simulink model "servo"  (R2018a)
settings: Solver=VariableStepAuto  StartTime=0.0  StopTime=T  RelTol=1e-3
values from neighbouring files (symbols this model uses):
  C0 = 0.024    [asserv_ge2M.m]
  f = 5.06e-5    (= 5.06e-05)    [asserv_ge2M.m]
  Ghelice = 28.35*h*D^3*10^-10*Sgouv    [asserv_ge2M.m]
  Gredu = 1    [asserv_ge2M.m]
  Gservo = 1    [asserv_ge2M.m]
  J = 8.3e-5    (= 8.3e-05)    [asserv_ge2M.m]
  Kphi = 0.127    [asserv_ge2M.m]
  KpS = 1    [asserv_ge2M.m]
  L = 2.2e-3    (= 0.0022)    [asserv_ge2M.m]
  R = 1.52    [asserv_ge2M.m]
  Step = pi    (= 3.14159265359)    [asserv_ge2M.m]
  Vit = 10000/60    (= 166.666666667)    [asserv_ge2M.m]
libraries: simulink x1
settings Model: Creator=xoxox  LastModifiedBy=xoxox

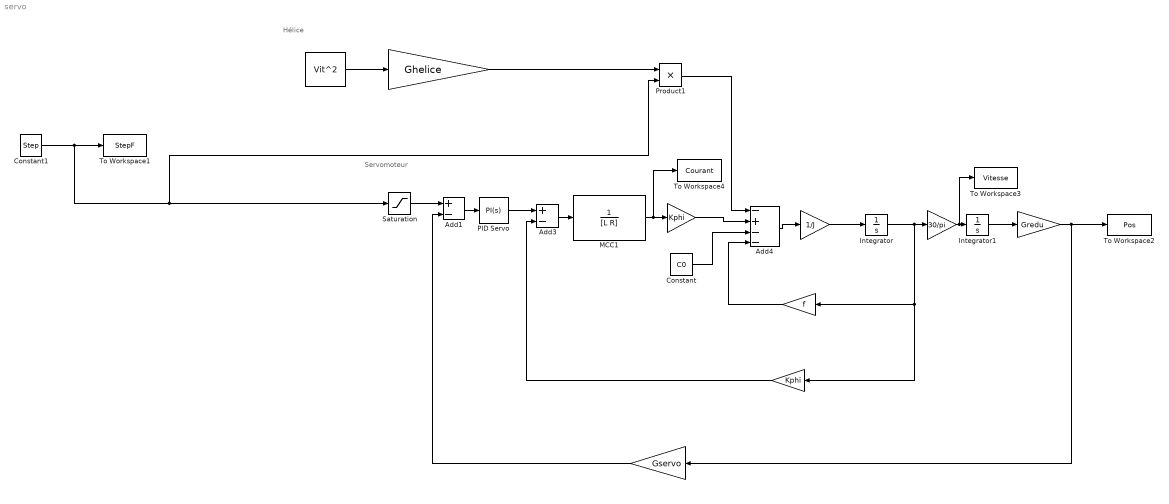
== system servo ==
  note: Servomoteur
  note: Hélice
  " " : Gain  Gain=Kphi
  " " : Gain  Gain=Gservo
  " " : Gain  Gain=Gredu
  "  " : Gain  Gain=Kphi
  " " : Constant  Value=Vit^2
  " " : Gain  Gain=1/J
  " " : Gain  Gain=Ghelice
  "     " : Gain  Gain=f
  " " : Gain  Gain=30/pi
  Add1 : Sum  Inputs=+-
  Add3 : Sum  Inputs=+-
  Add4 : Sum  Inputs=-+--
  Constant : Constant  Value=C0
  Constant1 : Constant  Value=Step
  Integrator : Integrator
  Integrator1 : Integrator
  MCC1 : TransferFcn  Denominator=[L R]
  PID Servo : simulink/Continuous/PID Controller  Controller=PI  TimeDomain=Continuous-time  SampleTime=-1  IntegratorMethod=Forward Euler  FilterMethod=Forward Euler  Form=Parallel  UseFilter=on  ControllerParametersSource=internal  P=KpS  I=0  D=0  N=100  InitialConditionSource=internal  InitialConditionForIntegrator=0  InitialConditionForFilter=0  ExternalReset=none  LimitOutput=off  UpperSaturationLimit=inf  LowerSaturationLimit=-inf  LinearizeAsGain=on  AntiWindupMode=none  Kb=1  TrackingMode=off  Kt=1  PParamMin=[]  PParamMax=[]  IParamMin=[]  IParamMax=[]  DParamMin=[]  DParamMax=[]  NParamMin=[]  NParamMax=[]  KbParamMin=[]  KbParamMax=[]  KtParamMin=[]  KtParamMax=[]  POutMin=[]  POutMax=[]  IOutMin=[]  IOutMax=[]  DOutMin=[]  DOutMax=[]  NOutMin=[]  NOutMax=[]  KbOutMin=[]  KbOutMax=[]  KtOutMin=[]  KtOutMax=[]  IntegratorOutMin=[]  IntegratorOutMax=[]  FilterOutMin=[]  FilterOutMax=[]  SumOutMin=[]  SumOutMax=[]  SumI1OutMin=[]  SumI1OutMax=[]  SumI2OutMin=[]  SumI2OutMax=[]  SumI3OutMin=[]  SumI3OutMax=[]  SumDOutMin=[]  SumDOutMax=[]  SaturationOutMin=[]  SaturationOutMax=[]  IntegratorContinuousStateAttributes=''  IntegratorStateMustResolveToSignalObject=off  IntegratorRTWStateStorageClass=Auto  FilterContinuousStateAttributes=''  FilterStateMustResolveToSignalObject=off  FilterRTWStateStorageClass=Auto  DifferentiatorICPrevScaledInput=0  DifferentiatorOutMin=[]  DifferentiatorOutMax=[]  FilterDiffOutCoefMin=[]  FilterDiffOutCoefMax=[]  SumDenOutMin=[]  SumDenOutMax=[]  SumNumOutMin=[]  SumNumOutMax=[]  ReciprocalOutMin=[]  ReciprocalOutMax=[]  DivideOutMin=[]  DivideOutMax=[]  TunerSelectOption=Transfer Function Based (PID Tuner App)
  Product1 : Product
  Saturation : Saturate  UpperLimit=pi  LowerLimit=-pi
  To Workspace1 : ToWorkspace  VariableName=StepF  SaveFormat=Timeseries  SampleTime=-1
  To Workspace2 : ToWorkspace  VariableName=Pos  SaveFormat=Timeseries  SampleTime=-1
  To Workspace3 : ToWorkspace  VariableName=Vitesse  SaveFormat=Timeseries  SampleTime=-1
  To Workspace4 : ToWorkspace  VariableName=Courant  SaveFormat=Timeseries  SampleTime=-1
  wires:
  Add3/1 -> MCC1/1
  MCC1/1 -> To Workspace4/1, "  "/1
  Integrator/1 -> "     "/1, " "/1, " "/1
  " "/1 -> To Workspace3/1, Integrator1/1
  " "/1 -> Add3/2
  " "/1 -> Integrator/1
  Add4/1 -> " "/1
  Integrator1/1 -> " "/1
  PID Servo/1 -> Add3/1
  Add1/1 -> PID Servo/1
  " "/1 -> Add1/2
  " "/1 -> " "/1, To Workspace2/1
  Saturation/1 -> Add1/1
  " "/1 -> Product1/1
  " "/1 -> " "/1
  Constant1/1 -> Product1/2, Saturation/1, To Workspace1/1
  "     "/1 -> Add4/4
  Constant/1 -> Add4/3
  "  "/1 -> Add4/2
  Product1/1 -> Add4/1
